simulink model "fuera_de_linea"  (Simulink 5.0)
settings: Solver=ode45  StartTime=0.0  StopTime=10.0  RelTol=1e-3
undefined symbols (not defined in the file): ts
settings Model: LastModifiedBy=pc1

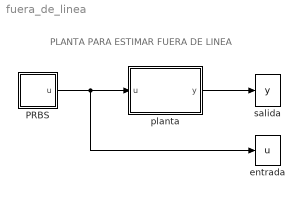
== system fuera_de_linea ==
  note: PLANTA PARA ESTIMAR FUERA DE LINEA
  PRBS : Subsystem
  entrada : ToWorkspace  VariableName=u  SampleTime=-1  SaveFormat=Array
  planta : Subsystem
  salida : ToWorkspace  VariableName=y  SampleTime=-1  SaveFormat=Array
  wires:
  PRBS/1(u) -> entrada/1, planta/1(u)
  planta/1(y) -> salida/1

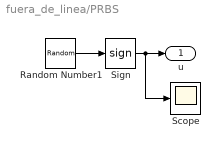
== system fuera_de_linea/PRBS ==
  Random Number1 : RandomNumber  SampleTime=0
  Scope : Scope
  Sign : Signum
  u : Outport
  wires:
  Random Number1/1 -> Sign/1
  Sign/1 -> u/1, Scope/1

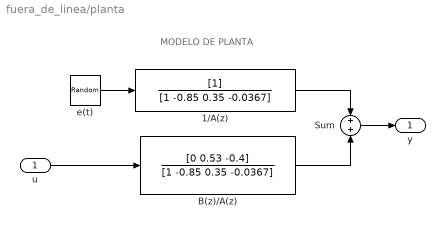
== system fuera_de_linea/planta ==
  note: MODELO DE PLANTA
  u : Inport
  1/A(z) : DiscreteFilter  Denominator=[1 -0.85 0.35 -0.0367]  SampleTime=ts
  B(z)/A(z) : DiscreteFilter  Numerator=[0 0.53 -0.4]  Denominator=[1 -0.85 0.35 -0.0367]  SampleTime=ts
  Sum : Sum  SaturateOnIntegerOverflow=on
  e(t) : RandomNumber  Variance=0.001  SampleTime=ts
  y : Outport
  wires:
  e(t)/1 -> 1/A(z)/1
  u/1 -> B(z)/A(z)/1
  Sum/1 -> y/1
  1/A(z)/1 -> Sum/1
  B(z)/A(z)/1 -> Sum/2
